simulink library "target_gen_lib"  (R2018b)
settings: Solver=VariableStepAuto  StartTime=0.0  StopTime=10.0  RelTol=1e-3
undefined symbols (not defined in the file): fswParams
libraries: sharedtransform x1, vrlib x1, quat_rectify_lib x1
settings Model: Creator=colem  LastModifiedBy=Taylor

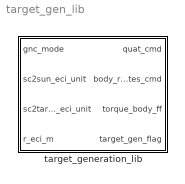
== system target_gen_lib ==
  target_generation_lib : Subsystem  TreatAsAtomicUnit=on
      settings: RTWFcnNameOpts=Use subsystem name  RTWFileNameOpts=Use subsystem name

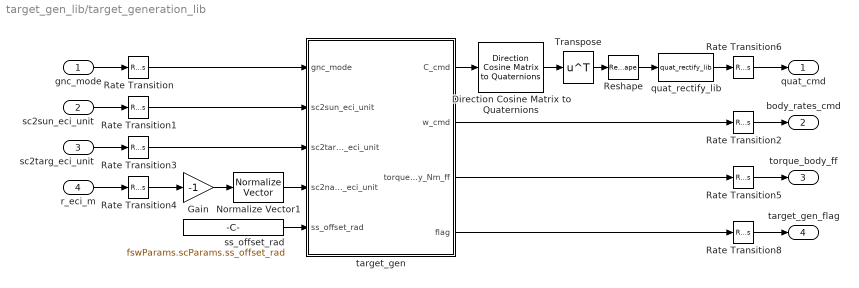
== system target_gen_lib/target_generation_lib ==
  gnc_mode : Inport
  sc2sun_eci_unit : Inport  Port=2
  sc2targ_eci_unit : Inport  Port=3
  r_eci_m : Inport  Port=4
  Direction Cosine Matrix to Quaternions : sharedtransform/Direction Cosine Matrix  to Quaternions  aMode=0  action=Warning  tolerance=1e-12
      settings: SourceProductName=Aerospace Blockset  SourceProductBaseCode=AE
  Gain : Gain  Gain=-1
  Normalize Vector1 : vrlib/Utilities/Normalize Vector  maxzero=0
      settings: SourceProductName=Simulink 3D Animation  SourceProductBaseCode=VR
  Rate Transition : RateTransition  InitialCondition=fswParams.mode_select.gnc_mode_ic  OutPortSampleTime=fswParams.sample_time_s
  Rate Transition1 : RateTransition  OutPortSampleTime=fswParams.sample_time_s
  Rate Transition2 : RateTransition
  Rate Transition3 : RateTransition  OutPortSampleTime=fswParams.sample_time_s
  Rate Transition4 : RateTransition  OutPortSampleTime=fswParams.sample_time_s
  Rate Transition5 : RateTransition
  Rate Transition6 : RateTransition  InitialCondition=fswParams.controllers.reorientation.qd
  Rate Transition8 : RateTransition
  Reshape : Reshape
  Transpose : Math  Operator=transpose  SaturateOnIntegerOverflow=on
  quat_rectify_lib : quat_rectify_lib/quat_rectify_lib
  ss_offset_rad : Constant  Value=fswParams.scParams.ss_offset_rad
  target_gen : MATLAB Function  TreatAsAtomicUnit=on
  quat_cmd : Outport
  body_rates_cmd : Outport  Port=2
  torque_body_ff : Outport  Port=3
  target_gen_flag : Outport  Port=4
  wires:
  Rate Transition8/1 -> target_gen_flag/1
  sc2targ_eci_unit/1 -> Rate Transition3/1
  target_gen/4(flag) -> Rate Transition8/1
  gnc_mode/1 -> Rate Transition/1
  sc2sun_eci_unit/1 -> Rate Transition1/1
  Transpose/1 -> Reshape/1
  Rate Transition6/1 -> quat_cmd/1
  r_eci_m/1 -> Rate Transition4/1
  Gain/1 -> Normalize Vector1/1
  Normalize Vector1/1 -> target_gen/4(sc2nadir_eci_unit)
  Rate Transition1/1 -> target_gen/2(sc2sun_eci_unit)
  Rate Transition/1 -> target_gen/1(gnc_mode)
  Rate Transition3/1 -> target_gen/3(sc2targ_eci_unit)
  Rate Transition4/1 -> Gain/1
  ss_offset_rad/1 -> target_gen/5(ss_offset_rad)
  target_gen/2(w_cmd) -> Rate Transition2/1
  Rate Transition2/1 -> body_rates_cmd/1
  target_gen/3(torque_body_Nm_ff) -> Rate Transition5/1
  Rate Transition5/1 -> torque_body_ff/1
  target_gen/1(C_cmd) -> Direction Cosine Matrix to Quaternions/1
  Direction Cosine Matrix to Quaternions/1 -> Transpose/1
  Reshape/1 -> quat_rectify_lib/1
  quat_rectify_lib/1 -> Rate Transition6/1

== matlab function target_gen_lib/target_generation_lib/target_gen ==
  data: gnc_mode input size=1; C_cmd output double size=[3 3]; w_cmd output double size=3; torque_body_Nm_ff output double size=3; sc2sun_eci_unit input size=3; sc2targ_eci_unit input size=3; sc2nadir_eci_unit input; flag output uint8 size=1; ss_offset_rad input
function [C_cmd,w_cmd,torque_body_Nm_ff,flag] = target_gen(gnc_mode, ...
        sc2sun_eci_unit, sc2targ_eci_unit, sc2nadir_eci_unit, ss_offset_rad)
%TARGET_GEN FSW Target Generation Library
%
% Possible GNC modes for SOC-i:
%   CLPM        = 0
%   LPM         = 1
%   Idle        = 2
%   ASM         = 3
%   Desat       = 4
%   SunSeek     = 5
%   Nominal     = 6
%   Imaging     = 7
%   SOAR        = 8
%
% Cole Morgan | T. P. Reynolds
%#codegen

% Body frame vector definitions
COM     = [  0.0;  0.0;  1.0  ]; % COM antenna boresight vector (F_body)
IMG     = [  0.0;  0.0; -1.0  ]; % image camera boresight vector (F_body)
SP      = [  0.0;  1.0;  0.0  ]; % sun sensor boresight vector (F_body)

% Rotate the SP vector into the target frame using ss_offset_rad
flag    = uint8(0);
tol     = 1e-3;         % parallel vector tolerance
soff    = sin(ss_offset_rad);
coff    = cos(ss_offset_rad);
C_B2T   = [ coff, soff, 0.0; -soff, coff, 0.0; 0.0, 0.0, 1.0 ]; 

% Target frame definitions (if different from body frame)
SP_T = C_B2T * SP;

% Uncomment for testing only %   
% SP      = [1;3;0];
% -------------------------- %

% Nominal angular rate command
w_cmd = zeros(3,1);

% Nominal feedforward torque command
torque_body_Nm_ff = zeros(3,1);

% Validity Checks
if (norm(sc2sun_eci_unit) < tol) 
    C_cmd   = eye(3);
    flag    = uint8(1);
    return;
elseif (norm(sc2targ_eci_unit) < tol)
    C_cmd   = eye(3);
    flag    = uint8(2);
    return;
elseif (norm(sc2nadir_eci_unit) < tol)
    C_cmd   = eye(3);
    flag    = uint8(3);
    return;
end

% Main Code
if ( gnc_mode == 7 )
    % primary   : align the camera boresight with the target direction
    % secondary : align offset sun sensor boresight with inertial sun
    %             direction
    if ( abs(dot(sc2sun_eci_unit,sc2targ_eci_unit)) > 1-tol )
        C_cmd   = eye(3);
        flag    = uint8(4);
        return;
    end
    C_cmd = align_vecs(SP_T, sc2sun_eci_unit, IMG, sc2targ_eci_unit);
        
elseif ( (gnc_mode == 4 || gnc_mode == 5 || gnc_mode == 6) )
    % primary   : align offset sun sensor boresight with inertial sun
    %             direction
    % secondary : align the antenna boresight with the nadir direction
    if ( abs(dot(sc2nadir_eci_unit,sc2sun_eci_unit)) > 1-tol )           
        C_cmd   = eye(3);
        flag    = uint8(5);
        return;
    end
    C_cmd = align_vecs(SP_T, sc2sun_eci_unit, COM, sc2nadir_eci_unit);

else
    % No attitude commanded from here for CLPM, LPM, Idle, ASM & SOAR modes
    C_cmd   = eye(3);
    
end

end

function [C_cmd] = align_vecs(Body1, Inertial1, Body2, Inertial2) 
    
    % Body
    Body1 = Body1./norm(Body1); %takes precident
    Body2 = Body2./norm(Body2);
    Xtb = Body1;
    Ytb = cross(Body1,Body2);
    Ytb = Ytb./norm(Ytb);%/norm(cross(Body1,Body2));
    Ztb = cross(Body1,Ytb);
    Ztb = Ztb./norm(Ztb);%/norm(cross(Body1,Ytb));
    
    % Inertial
    Inertial1 = Inertial1./norm(Inertial1); % set to align with B1
    Inertial2 = Inertial2./norm(Inertial2); % set to partially align with B2
    Xti = Inertial1;
    Yti = cross(Inertial1,Inertial2);
    Yti = Yti./norm(Yti);%/norm(cross(Inertial1,Inertial2));
    Zti = cross(Inertial1,Yti);
    Zti = Zti./norm(Zti);%/norm(cross(Inertial1,Yti));
    
    % Stack vectors
    Cb  = [Xtb, Ytb, Ztb];
    Ci  = [Xti, Yti, Zti];
    
    % Commanded DCM ( body to inertial )
    C_cmd   = Cb*Ci';

end
